simulink model "enabled_subsystem"  (R2024b)
settings: Solver=VariableStepAuto  StartTime=0.0  StopTime=10.0  RelTol=1e-3
settings Model: Creator=balaj  LastModifiedBy=balaj

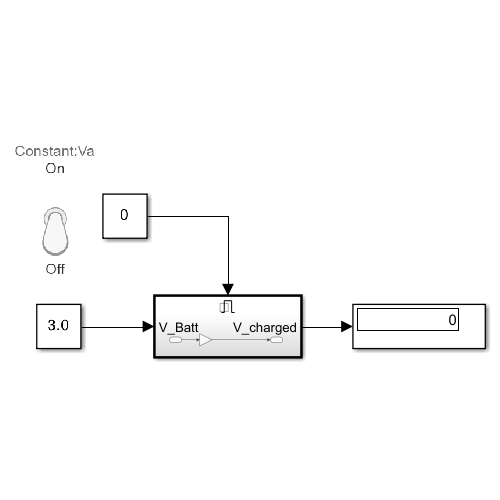
[thumbnail: Simulink's stored preview of the top-level diagram]
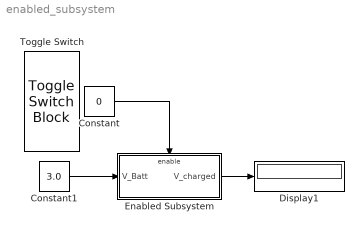
== system enabled_subsystem ==
  Constant : Constant  Value=0
  Constant1 : Constant  Value=3.0
  Display1 : Display
  Enabled Subsystem : Subsystem  TreatAsAtomicUnit=on
  Toggle Switch : ToggleSwitchBlock
      settings: Values={{'Off', 'On'}, [0 1]}
  wires:
  Constant/1 -> Enabled Subsystem/Enable
  Constant1/1 -> Enabled Subsystem/1(V_Batt)
  Enabled Subsystem/1(V_charged) -> Display1/1

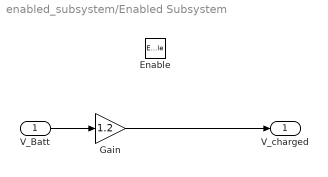
== system enabled_subsystem/Enabled Subsystem ==
  V_Batt : Inport
  Enable : EnablePort
  Gain : Gain  Gain=1.2
  V_charged : Outport
  wires:
  V_Batt/1 -> Gain/1
  Gain/1 -> V_charged/1
